simulink model "Ball_and_Plate_MicroLabBox_student"  (R2019b)
settings: Solver=ode1  StartTime=0.0  StopTime=Inf  FixedStep=0.001  RelTol=1e-3
PostLoadFcn:
  | , if any(exist('dsrtsu_mdlpostloadfcn', 'file') ~= 0), dsrtsu_mdlpostloadfcn('Execute', bdroot); end,
InitFcn:
  | , if any(exist('rtifpga_mdlclblib', 'file') ~= 0), rtifpga_mdlclblib('Init', bdroot); end,
undefined symbols (not defined in the file): A_obs, A_robust, B_obs, B_robust, ball_pos_sat, ball_vel_sat, C_obs, C_robust, D_obs, D_robust, g, K_lqr, path, plate_angle_sat, Q_kf, R_kf, Ts_fast, Ts_Inner, Ts_Outer, uA, uB, uC
libraries: rtiemclib x6, simulink x3, rtiethernetlib x3, rti1202lib_dac_class1 x3, mpclib x1
(part 1 of 3)
Description:
  | Standard RTI1202 template.
  | Supported MATLAB version:  R2019b.
settings Model: Tag=RTI1202  DSRTSU_INTERNAL_RTI_VER=570  DSRTSU_INTERNAL_RTI_TYPE=rti1202  RTICANMMDATA=struct('GeneralSetupData',struct('modelroot','C:\git\SystemsAndControlIntegrationProject_5SC25\Experiment\BallANDPlate','generalsettings',struct('filesettings',struct('destfolder',struct('Name','RTICANMM_FILES','Check',1),'buildfolder',struct('Name','.','Check',1),'AbsDestfolder',struct('Name','C:\git\SystemsAndControlIntegrationProject_5SC25\Experiment\BallANDPlate\RTICANMM_FILES'),'AbsBuildfolder',struct('Name','C:\git\SystemsAndControlIntegrationProject_5SC25\Experiment\BallANDPlate'))),'options',struct('addpaths',1,'rmpaths',1,'addtrcexclusion',true,'cannavigator',struct('checkmonitoring',0),'show_usrtrc',0,'use_usrtrc',0),'advanced',struct('options',ones(1,100)),'MPSetup',{{}},'RTI',struct('Type','RTI1202','Ver','7.15','Date','02-Nov-2020'),'modelname','Ball_and_Plate_MicroLabBox_student','block','Ball_and_Plate_MicroLabBox_student'))  DSRTSU_INTERNAL_RTIFPGA=170  Creator=20201603  LastModifiedBy=20242496
settings DataIOCC: ReturnWorkspaceOutputs=off
settings OptimizationCC: BlockReduction=off  OptimizeBlockIOStorage=off  BufferReuse=off  GlobalBufferReuse=off  ExpressionFolding=off  LocalBlockOutputs=off  OptimizeDataStoreBuffers=off  BusAssignmentInplaceUpdate=off
settings DebuggingCC: PregeneratedLibrarySubsystemCodeDiagnostic=none  ArithmeticOperatorsInVariantConditions=warning
settings HardwareCC: ProdBitPerPointer=32  ProdBitPerSizeT=32  ProdBitPerPtrDiffT=32  ProdLargestAtomicInteger=Integer  ProdEndianess=BigEndian  ProdWordSize=32  ProdLongLongMode=on  ProdHWDeviceType=Custom Processor->Custom  TargetIntDivRoundTo=Zero  TargetEndianess=BigEndian  TargetHWDeviceType=Custom Processor->Custom
settings ModelReferenceCC: EnableParallelModelReferenceBuilds=on  ParallelModelReferenceMATLABWorkerInit=Load Top Model
settings SFSimCC: SimUseLocalCustomCode=off  MATLABDynamicMemAlloc=off  CustomCodeUndefinedFunction=UseInterfaceOnly
settings RTWCC: Description=dSPACE DS1202 Hardware Platform  SystemTargetFile=rti1202.tlc  MakeCommand=make_rti  TemplateMakefile=rti1202.tmf  RTWUseLocalCustomCode=off
settings CodeAppCC: StateflowObjectComments=on
settings STFCustomTargetCC: ParMdlRefBuildCompliant=on  SystemTargetFile=rti1202.tlc
settings GRTTargetCC: TargetLangStandard=C89/C90 (ANSI)  CompOptLevelCompliant=off  ConcurrentExecutionCompliant=off  CombineOutputUpdateFcns=off  MatFileLogging=off  CPPClassGenCompliant=off  UseToolchainInfoCompliant=off
settings ConfigComp: CovMetricSettings=dswe

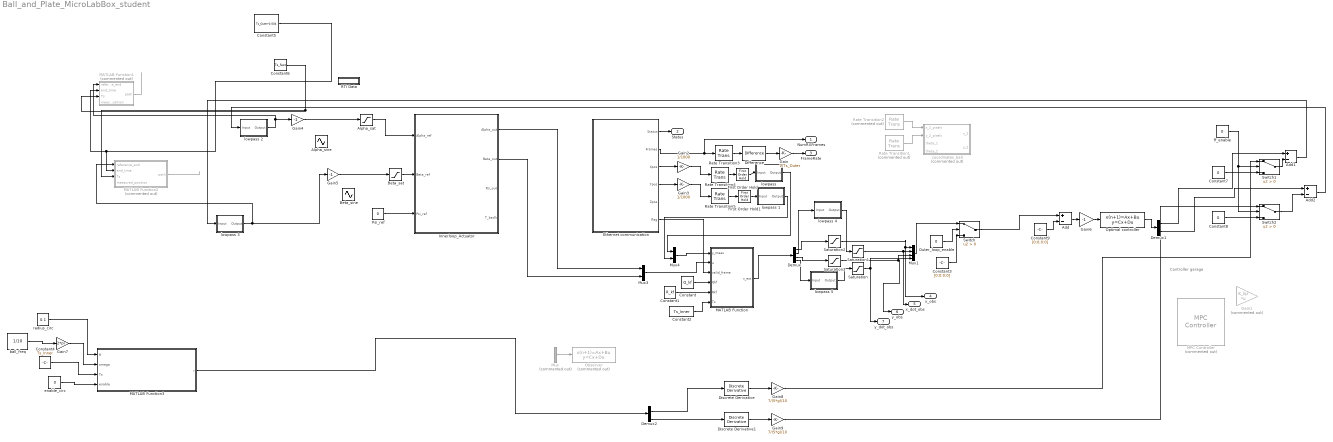
== system Ball_and_Plate_MicroLabBox_student ==
  note: Controller garage
  Add : Sum  Inputs=+-
  Add1 : Sum  Inputs=+-
  Add2 : Sum  Inputs=+-
  "Alpha_sat " : Saturate  UpperLimit=plate_angle_sat  LowerLimit=-plate_angle_sat
  "Alpha_sine " : Sin  Amplitude=0.01  SampleTime=0
  "Beta_sat " : Saturate  UpperLimit=plate_angle_sat  LowerLimit=-plate_angle_sat
  Beta_sine : Sin  Amplitude=0.01  SampleTime=0
  Constant : Constant  Value=Q_kf
  Constant1 : Constant  Value=R_kf
  Constant2 : Constant  Value=Ts_Inner
  Constant3 : Constant  Value=[0;0;0;0]
  Constant4 : Constant  Value=Ts_Inner
  Constant5 : Constant  Value=Ts_Outer-0.004
  Constant6 : Constant  Value=Ts_fast
  Constant7 : Constant  Value=0
  Constant8 : Constant  Value=0
  Constant9 : Constant  Value=[0;0;0;0]
  Demux : Demux
  Demux1 : Demux  Outputs=2
  Demux2 : Demux
  Difference : simulink/Discrete/Difference  ICPrevInput=0  OutMin=[]  OutMax=[]  OutDataType=fixdt(1, 16)  OutScaling=2^-10  DoSatur=off
  Discrete Derivative : simulink/Discrete/Discrete Derivative  gainval=1.0  ICPrevScaledInput=0.0  OutMin=[]  OutMax=[]  OutDataType=fixdt(1, 16)  OutScaling=2^-10  DoSatur=off
  Discrete Derivative1 : simulink/Discrete/Discrete Derivative  gainval=1.0  ICPrevScaledInput=0.0  OutMin=[]  OutMax=[]  OutDataType=fixdt(1, 16)  OutScaling=2^-10  DoSatur=off
  Ethernet communication : Subsystem
  First Order Hold : FirstOrderHold  ErrorTolerance=inf
  First Order Hold1 : FirstOrderHold  ErrorTolerance=inf
  Gain : Gain  Gain=1/Ts_Outer
  Gain1 : Gain  Commented=on  Gain=K_lqr  Multiplication=Matrix(K*u)
  Gain2 : Gain  Gain=1/1000
  Gain3 : Gain  Gain=1/1000
  Gain4 : Gain  Gain=-1
  Gain5 : Gain  Gain=-1
  Gain6 : Gain  Gain=-1
  Gain7 : Gain  Gain=2*pi
  Gain8 : Gain  Gain=7/(5*g)/10
  Gain9 : Gain  Gain=7/(5*g)/10
  Innerloop_Actuator : Subsystem
  MATLAB Function : MATLAB Function  TreatAsAtomicUnit=on
  MATLAB Function1 : MATLAB Function  Commented=on  TreatAsAtomicUnit=on
  MATLAB Function2 : MATLAB Function  Commented=on  TreatAsAtomicUnit=on
  MATLAB Function3 : MATLAB Function  TreatAsAtomicUnit=on
  MPC Controller : mpclib/MPC Controller  Commented=on  SCDEnableBlockLinearizationSpecification=on  mpcobj=mpcobj  is_multiple=0  enable_value=0  return_u0=off  updateMPCinCallerWorkspace=on  md_inport=off  mv_inport=off  uref_inport=off  return_cost=off  return_mvseq=off  return_qpstatus=off  return_xseq=off  return_state=off  return_ovseq=off  state_inport=on  umin_inport=off  umax_inport=off  ymin_inport=off  ymax_inport=off  cc_inport=off  ywt_inport=off  uwt_inport=off  duwt_inport=off  rhoeps_inport=off  pm_inport=off  MaximumP=10  HorizonChoice=FixedHorizon  n_ts=0.02  n_p=25  n_mv=2  n_md=0  n_ud=0  n_mo=4  n_uo=0  BlockDataType=double  SampleTimeInherited=off  switch_inport=off
  Mux : Mux  Commented=on
  Mux1 : Mux
  Mux3 : Mux  Inputs=2
  Mux4 : Mux  Inputs=2
  "Observer " : DiscreteStateSpace  Commented=on  A=A_obs  B=B_obs  C=C_obs  D=D_obs  SampleTime=Ts_Outer
  Optimal controller : DiscreteStateSpace  A=A_robust  B=B_robust  C=C_robust  D=D_robust  SampleTime=Ts_Inner
  Outer_loop_enable : Constant  Value=0
  "Psi_ref " : Constant  Value=0
  RTI Data : Subsystem  Tag=struct('RTIDataServer',struct('RTIDataServerVs','2','RTIModelDescription','struct(''main'',''Ball_and_Plate_MicroLabBox_student'',''sub'','''',''isMp'',0)'))  LoadFcn="if exist('rtidc'), try,  rtidc('DataHostBlockClbLoad', gcbh); catch, disp(['Warning: ''LoadFcn'' for RTI Data block failed: ' lasterr]); end, end,"  mask(RTI_DATA_HOST){}
      mask help:
      | RTI Data Block.
      | This block is used by RTI to store internal model-dependent data.
      | Please keep this block on the root level of the model. Deleting this block will result in data loss.
      |
      | NEVER DELETE OR COPY THIS BLOCK!
      settings: CopyFcn="if exist('rtidc'), try,  rtidc('DataHostBlockClbCopy', gcbh); catch, disp(['Warning: ''CopyFcn'' for RTI Data block failed: ' lasterr]); end, end,"  DeleteFcn="if exist('rtidc'), try,  rtidc('DataHostBlockClbDelete', gcbh); catch, disp(['Warning: ''DeleteFcn'' for RTI Data block failed: ' lasterr]); end, end,"  ModelCloseFcn="if exist('rtidc'), try,  rtidc('DataHostBlockClbModelClose', gcbh); catch, disp(['Warning: ''ModelCloseFcn'' for RTI Data block failed: ' lasterr]); end, end,"  PreSaveFcn="if exist('rtidc'), try,  rtidc('DataHostBlockClbPreSave', gcbh); catch, disp(['Warning: ''PreSaveFcn'' for RTI Data block failed: ' lasterr]); end, end,"  PostSaveFcn="if exist('rtidc'), try,  rtidc('DataHostBlockClbPostSave', gcbh); catch, disp(['Warning: ''PostSaveFcn'' for RTI Data block failed: ' lasterr]); end, end,"  NameChangeFcn="if exist('rtidc'), try,  rtidc('DataHostBlockClbNameChange', gcbh); catch, disp(['Warning: ''NameChangeFcn'' for RTI Data block failed: ' lasterr]); end, end,"
      mask Help:
      | RTI Data Block.
      | This block is used by RTI to store internal model-dependent data.
      | Please keep this block on the root level of the model. Deleting this block will result in data loss.
      | 
      | NEVER DELETE OR COPY THIS BLOCK!
      mask Display:
      | text(0.5, 0.5, 'RTI Data', 'HorizontalAlignment', 'center');
      | plot([1 0]);
  Rate Transition1 : RateTransition  Commented=on  Deterministic=off  OutPortSampleTimeMultiple=Ts_Outer  OutPortSampleTime=Ts_Outer
  Rate Transition2 : RateTransition  Commented=on  Deterministic=off  OutPortSampleTimeMultiple=Ts_Outer  OutPortSampleTime=Ts_Outer
  Rate Transition3 : RateTransition  Deterministic=off  OutPortSampleTimeMultiple=Ts_Outer  OutPortSampleTime=Ts_Outer
  Rate Transition4 : RateTransition  Deterministic=off  OutPortSampleTimeMultiple=Ts_Outer  OutPortSampleTime=Ts_Outer
  Rate Transition5 : RateTransition  Deterministic=off  OutPortSampleTimeMultiple=Ts_Outer  OutPortSampleTime=Ts_Outer
  Saturation : Saturate  UpperLimit=ball_vel_sat  LowerLimit=-ball_vel_sat
  Saturation1 : Saturate  UpperLimit=ball_vel_sat  LowerLimit=-ball_vel_sat
  Saturation2 : Saturate  UpperLimit=ball_pos_sat  LowerLimit=-ball_pos_sat
  Saturation3 : Saturate  UpperLimit=ball_pos_sat  LowerLimit=-ball_pos_sat
  Switch : Switch  Criteria=u2 > Threshold
  Switch1 : Switch  Criteria=u2 > Threshold
  Switch2 : Switch  Criteria=u2 > Threshold
  ball_freq : Constant  Value=1/10
  coordinates_ball : MATLAB Function  Commented=on  TreatAsAtomicUnit=on
  enable_circ : Constant  Value=0
  ff_enable : Constant  Value=0
  "lowpass " : Subsystem
  lowpass 1 : Subsystem
  lowpass 2 : Subsystem
  lowpass 3 : Subsystem
  lowpass 4 : Subsystem
  lowpass 5 : Subsystem
  radius_circ : Constant  Value=0.1
  NumRXFrames : Outport
  Status : Outport  Port=2
  "FrameRate " : Outport  Port=3
  x_obs : Outport  Port=4
  x_dot_obs : Outport  Port=5
  y_obs : Outport  Port=6
  y_dot_obs : Outport  Port=7
  wires:
  Ethernet communication/2("Frames ") -> NumRXFrames/1, Rate Transition3/1
  Rate Transition3/1 -> Difference/1
  Difference/1 -> Gain/1
  Gain/1 -> "FrameRate "/1
  Ethernet communication/1("Status ") -> Status/1
  Rate Transition2/1 -> coordinates_ball/1(x_2_pixels)
  Rate Transition1/1 -> coordinates_ball/2(y_2_pixels)
  "Psi_ref "/1 -> Innerloop_Actuator/3("Psi_ref ")
  Innerloop_Actuator/1(Alpha_out) -> Mux3/1
  Innerloop_Actuator/2(Beta_out) -> Mux3/2
  Mux/1 -> "Observer "/1
  Demux/1 -> Saturation2/1
  Demux/4 -> lowpass 5/1(Input)
  Demux/3 -> Saturation3/1
  Demux/2 -> lowpass 4/1(Input)
  Saturation/1 -> Mux1/4, y_dot_obs/1
  Saturation1/1 -> Mux1/2, x_dot_obs/1
  Mux1/1 -> Switch/1
  Outer_loop_enable/1 -> Switch/2
  Constant3/1 -> Switch/3
  Add1/1 -> lowpass 3/1(Input)
  Add2/1 -> lowpass 2/1(Input)
  "Alpha_sat "/1 -> Innerloop_Actuator/1("Alpha_ref ")
  "Beta_sat "/1 -> Innerloop_Actuator/2("Beta_ref ")
  Ethernet communication/3("Xpos ") -> Gain2/1
  Ethernet communication/4("Ypos ") -> Gain3/1
  Rate Transition4/1 -> First Order Hold/1
  Rate Transition5/1 -> First Order Hold1/1
  Mux3/1 -> MATLAB Function/2(u)
  Mux4/1 -> MATLAB Function/1(y_meas)
  Ethernet communication/6(flag) -> MATLAB Function/3(valid_frame)
  Constant/1 -> MATLAB Function/4(Qkf)
  Constant1/1 -> MATLAB Function/5(Rkf)
  Constant2/1 -> MATLAB Function/6(Ts)
  Gain2/1 -> Rate Transition4/1
  Gain3/1 -> Rate Transition5/1
  "lowpass "/1(Output) -> Mux4/1
  lowpass 1/1(Output) -> Mux4/2
  Gain4/1 -> "Alpha_sat "/1
  Gain5/1 -> "Beta_sat "/1
  Constant5/1 -> MATLAB Function2/2(end_time), MATLAB Function1/2(end_time)
  Constant6/1 -> MATLAB Function2/3(Ts), MATLAB Function1/3(Ts)
  MATLAB Function1/1(path) -> ?
  MATLAB Function2/1(path) -> ?
  lowpass 2/1(Output) -> Gain4/1, MATLAB Function1/1(reference_end)
  lowpass 3/1(Output) -> Gain5/1, MATLAB Function2/1(reference_end)
  lowpass 4/1(Output) -> Saturation1/1
  lowpass 5/1(Output) -> Saturation/1
  Saturation2/1 -> Mux1/1, x_obs/1
  Saturation3/1 -> Mux1/3, y_obs/1
  Switch/1 -> Add/1
  MATLAB Function/1(x_est) -> Demux/1
  First Order Hold/1 -> "lowpass "/1(Input)
  First Order Hold1/1 -> lowpass 1/1(Input)
  Constant4/1 -> MATLAB Function3/3(Ts)
  radius_circ/1 -> MATLAB Function3/1(R)
  ball_freq/1 -> Gain7/1
  Gain7/1 -> MATLAB Function3/2(omega)
  enable_circ/1 -> MATLAB Function3/4(enable)
  MATLAB Function3/1(r) -> Demux2/1
  Demux2/2 -> Discrete Derivative/1
  Demux2/4 -> Discrete Derivative1/1
  Discrete Derivative1/1 -> Gain9/1
  Discrete Derivative/1 -> Gain8/1
  Gain8/1 -> Switch1/1
  Gain9/1 -> Switch2/1
  Demux1/1 -> Add1/1
  Demux1/2 -> Add2/1
  Switch1/1 -> Add1/2
  ff_enable/1 -> Switch2/2, Switch1/2
  Switch2/1 -> Add2/2
  Constant7/1 -> Switch1/3
  Constant8/1 -> Switch2/3
  Constant9/1 -> Add/2
  Add/1 -> Gain6/1
  Optimal controller/1 -> Demux1/1
  Gain6/1 -> Optimal controller/1

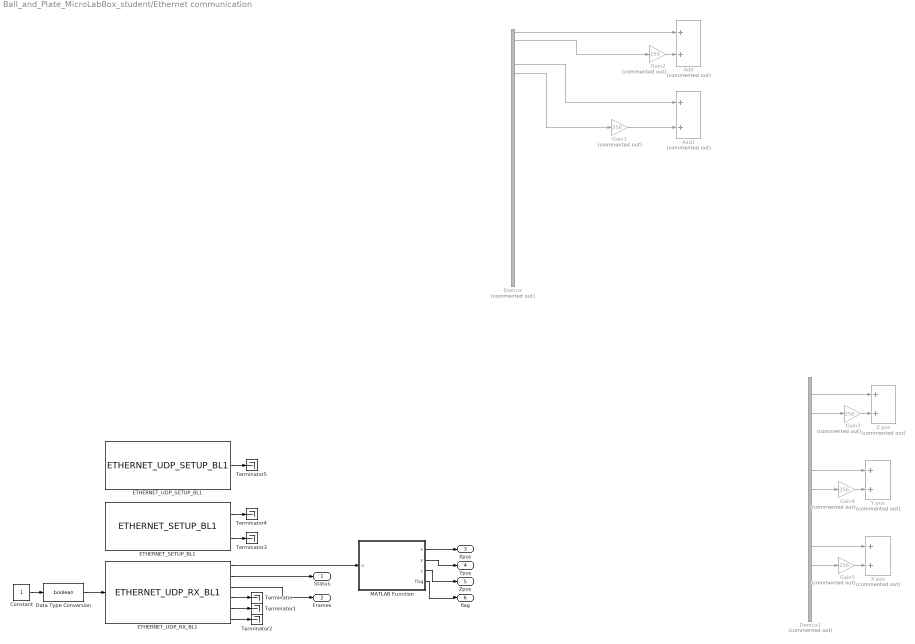
== system Ball_and_Plate_MicroLabBox_student/Ethernet communication ==
  " X pos" : Sum  Commented=on  AccumDataTypeStr=uint16
  Add : Sum  Commented=on  AccumDataTypeStr=uint16
  Add1 : Sum  Commented=on
  Constant : Constant
  Data Type Conversion : DataTypeConversion  OutDataTypeStr=boolean
  Demux : Demux  Commented=on  Outputs=32
  Demux1 : Demux  Commented=on  Outputs=12
  ETHERNET_SETUP_BL1 : rtiethernetlib/ETHERNET_SETUP_BL1  DSProperties=struct('RTI',struct('Version',uint32(2),'BlockType',struct('isSLSource',uint8(0),'isSLSink',uint8(0),'isHWSource',uint8(0),'isHWSink',uint8(0),'isSetup',uint8(1),'isInline',uint8(1),'isNonInline',uint8(0),'isInterrupt',uint8(0),'isChannelwise',uint8(0)),'IOBoardType','DSETHERNET','UnitType','ETHERNET','Identifier','SETUP','DialogType','ML','BlockSet','RTIETHERNET','SlaveProcessor','NONE'))  RTIBlockInterface=struct('OutputPortsWidth',int32([3 1 1 4]),'OutputPortsActive',[1 0 0 1],'OutputPortsName',{{['Link Status'],['Watchdog Status'],['DHCP Status'],['Local IP']}},'OutputPortsDataType',{{'SS_UINT32','SS_UINT32','SS_UINT32','SS_UINT8'}},'InitLevel',3,'IconTransparency','on','BlockDisplay',{{['Ethernet Setup\n\nLocal IP: 192.168.140.8'],'left'}},'DialogFcn','rtiethernetsetupgui','BlockName',struct('Token',{{'ETHERNET_SETUP_BL1'}}))  RTIBlockParameters=struct('DHCPserverMode',{{0,'OFF',[0 1]}},'LocalIpNum1',{{'192','OFF',[0 255]}},'LocalIpNum2',{{'168','OFF',[0 255]}},'LocalIpNum3',{{'140','OFF',[0 255]}},'LocalIpNum4',{{'8','OFF',[0 255]}},'SubnetMaskNum1',{{'255','OFF',[0 255]}},'SubnetMaskNum2',{{'255','OFF',[0 255]}},'SubnetMaskNum3',{{'255','OFF',[0 255]}},'SubnetMaskNum4',{{'0','OFF',[0 255]}},'GatewayNum1',{{'0','OFF',[0 255]}},'GatewayNum2',{{'0','OFF',[0 255]}},'GatewayNum3',{{'0','OFF',[0 255]}},'GatewayNum4',{{'0','OFF',[0 255]}},'LinkStatusOutPortMode',{{1,'OFF',[0 1]}},'NumOfEthConnectors',{{3,'ON',[1 16]}},'WatchdogStatusOutPortMode',{{0,'OFF',[0 1]}},'LocalIpOutPortMode',{{1,'OFF',[0 1]}},'IpAndSubmaskCheck',{{int32(1),'OFF',[0 1]}},'TLCFileName',{{'rtiethernetsetup','OFF',[]}})  RTISFcnParameters=struct('DHCPserverMode','int32','LocalIpNum1','uint8','LocalIpNum2','uint8','LocalIpNum3','uint8','LocalIpNum4','uint8','SubnetMaskNum1','uint8','SubnetMaskNum2','uint8','SubnetMaskNum3','uint8','SubnetMaskNum4','uint8','GatewayNum1','uint8','GatewayNum2','uint8','GatewayNum3','uint8','GatewayNum4','uint8','LinkStatusOutPortMode','int32','NumOfEthConnectors','int32','WatchdogStatusOutPortMode','int32','LocalIpOutPortMode','int32','TLCFileName','char')  RTIBlockParaDefault=struct('DHCPserverMode',0,'LocalIpNum1',192,'LocalIpNum2',168,'LocalIpNum3',140,'LocalIpNum4',6,'SubnetMaskNum1',255,'SubnetMaskNum2',255,'SubnetMaskNum3',255,'SubnetMaskNum4',0,'GatewayNum1',0,'GatewayNum2',0,'GatewayNum3',0,'GatewayNum4',0,'LinkStatusOutPortMode',1,'NumOfEthConnectors',3,'WatchdogStatusOutPortMode',0,'LocalIpOutPortMode',0,'IpAndSubmaskCheck',1,'TLCFileName','rtiethernetsetup')
      settings: SourceProductName=dSPACE RTI Ethernet Blockset
  ETHERNET_UDP_RX_BL1 : rtiethernetlib/ETHERNET_UDP_RX_BL1  DSProperties=struct('RTI',struct('Version',uint32(1),'BlockType',struct('isSLSource',uint8(1),'isSLSink',uint8(1),'isHWSource',uint8(0),'isHWSink',uint8(1),'isSetup',uint8(0),'isInline',uint8(1),'isNonInline',uint8(0),'isInterrupt',uint8(0),'isChannelwise',uint8(0)),'IOBoardType','DSETHERNET','UnitType','UDP','Identifier','RXUDP','DialogType','ML','BlockSet','RTIETHERNET','SlaveProcessor','NONE'))  RTIBlockInterface=struct('OutputPortsWidth',int32([12 1 1 1 4 1]),'OutputPortsActive',[1 1 1 1 1 1],'OutputPortsName',{{'Data','Status',['Received Frames'],['Received Bytes'],['Remote IP'],['Remote Port']}},'OutputPortsDataType',{{'SS_UINT8','SS_UINT32','SS_DOUBLE','SS_UINT32','SS_UINT8','SS_UINT16'}},'InputPortsWidth',int32(1),'InputPortsActive',1,'InputPortsName',{{'Enable'}},'InputPortsDataType',{{'SS_BOOLEAN'}},'RWork',{{{'RECEIVED_FRAMES',uint32(1)}}},'InitLevel',3,'IconTransparency','on','BlockDisplay',{{['Ethernet UDP/IP\nRX\n\nSocket ID: 1'],'center'}},'DialogFcn','rtiethernetrxudpgui','BlockName',struct('Token',{{'ETHERNET_UDP_RX_BL1'}}))  RTIBlockParameters=struct('SocketIdIndex',{{2,'OFF',[1 2]}},'SocketId',{{1,'OFF',[-1 inf]}},'RemoteIp',{{['<NOT AVAILABLE>'],'OFF',[]}},'RemotePort',{{['<NOT AVAILABLE>'],'OFF',[]}},'LocalPort',{{49001,'OFF',[]}},'FrameSize',{{'12','OFF',[1 65507]}},'EnableVariableFrameSize',{{1,'OFF',[0 1]}},'VariableFrameSizeMode',{{1,'OFF',[1 2]}},'InterruptMode',{{0,'OFF',[0 1]}},'RemoteIpOutPortMode',{{1,'OFF',[0 1]}},'RemotePortOutPortMode',{{1,'OFF',[0 1]}},'TLCFileName',{{'rtiethernetrxudp','OFF',[]}})  RTISFcnParameters=struct('SocketIdIndex','int32','SocketId','double','FrameSize','uint16','EnableVariableFrameSize','int32','VariableFrameSizeMode','int32','InterruptMode','int32','RemoteIpOutPortMode','int32','RemotePortOutPortMode','int32','TLCFileName','char')  RTIBlockParaDefault=struct('SocketIdIndex',1,'SocketId',-1,'RemoteIp',['<NOT AVAILABLE>'],'RemotePort',['<NOT AVAILABLE>'],'LocalPort',['<NOT AVAILABLE>'],'FrameSize',1024,'EnableVariableFrameSize',0,'VariableFrameSizeMode',1,'InterruptMode',0,'RemoteIpOutPortMode',0,'RemotePortOutPortMode',0,'TLCFileName','rtiethernetrxudp')
      settings: SourceProductName=dSPACE RTI Ethernet Blockset
  ETHERNET_UDP_SETUP_BL1 : rtiethernetlib/ETHERNET_UDP_SETUP_BL1  DSProperties=struct('RTI',struct('Version',uint32(2),'BlockType',struct('isSLSource',uint8(1),'isSLSink',uint8(1),'isHWSource',uint8(0),'isHWSink',uint8(0),'isSetup',uint8(0),'isInline',uint8(1),'isNonInline',uint8(0),'isInterrupt',uint8(0),'isChannelwise',uint8(0)),'IOBoardType','DSETHERNET','UnitType','UDP','Identifier','SETUPUDP','DialogType','ML','BlockSet','RTIETHERNET','SlaveProcessor','NONE'))  RTIBlockInterface=struct('OutputPortsWidth',int32(2),'OutputPortsActive',1,'OutputPortsName',{{['RX Dropped Frames']}},'OutputPortsDataType',{{'SS_DOUBLE'}},'InputPortsWidth',int32([4 1]),'InputPortsActive',int32([0 0]),'InputPortsName',{{['RX Remote IP Filter'],['RX Remote Port Filter']}},'InputPortsDataType',{{'SS_UINT8','SS_UINT16'}},'RWork',{{{'RX_DROPPED_FRAMES',uint32(2)}}},'InitLevel',3,'IconTransparency','on','BlockDisplay',{{['Ethernet UDP/IP\nSetup\n\nSocket ID: 1'],'center'}},'DialogFcn','rtiethernetsetupudpgui','BlockName',struct('Token',{{'ETHERNET_UDP_SETUP_BL1'}}))  RTIBlockParameters=struct('SocketId',{{1,'OFF',[]}},'EnableSocketBind',{{1,'OFF',[0 1]}},'AcceptAnyRxRemoteIp',{{1,'OFF',[0 1]}},'RxRemoteIpNum1',{{'192','OFF',[0 255]}},'RxRemoteIpNum2',{{'168','OFF',[0 255]}},'RxRemoteIpNum3',{{'140','OFF',[0 255]}},'RxRemoteIpNum4',{{'100','OFF',[0 255]}},'EnableDynamicRxRemoteIpFilter',{{0,'OFF',[0 1]}},'AcceptAnyRxRemotePort',{{1,'OFF',[0 1]}},'RxRemotePort',{{'57272','OFF',[1 65535]}},'EnableDynamicRxRemotePortFilter',{{0,'OFF',[0 1]}},'TxRemoteIpNum1',{{'192','OFF',[0 255]}},'TxRemoteIpNum2',{{'168','OFF',[0 255]}},'TxRemoteIpNum3',{{'140','OFF',[0 255]}},'TxRemoteIpNum4',{{'100','OFF',[0 255]}},'TxRemotePort',{{'49002','OFF',[1 65535]}},'SpecifyLocalPort',{{1,'OFF',[0 1]}},'LocalPort',{{'49001','OFF',[1 65535]}},'InterruptMode',{{0,'OFF',[0 1]}},'RxDroppedFramesOutPortMode',{{1,'OFF',[0 1]}},'RemoteIpNumCheck',{{0,'OFF',[0 1]}},'RemotePortCheck',{{0,'OFF',[0 1]}},'LocalPortCheck',{{1,'OFF',[0 1]}},'DHCPserverModeEnabled',{{0,'OFF',[0 1]}},'TLCFileName',{{'rtiethernetsetupudp','OFF',[]}})  RTISFcnParameters=struct('SocketId','double','EnableSocketBind','int32','AcceptAnyRxRemoteIp','int32','RxRemoteIpNum1','uint8','RxRemoteIpNum2','uint8','RxRemoteIpNum3','uint8','RxRemoteIpNum4','uint8','EnableDynamicRxRemoteIpFilter','int32','AcceptAnyRxRemotePort','int32','RxRemotePort','uint16','EnableDynamicRxRemotePortFilter','int32','TxRemoteIpNum1','uint8','TxRemoteIpNum2','uint8','TxRemoteIpNum3','uint8','TxRemoteIpNum4','uint8','TxRemotePort','uint16','SpecifyLocalPort','int32','LocalPort','uint16','InterruptMode','int32','RxDroppedFramesOutPortMode','int32','DHCPserverModeEnabled','int32','TLCFileName','char')  RTIBlockParaDefault=struct('SocketId',-1,'EnableSocketBind',1,'AcceptAnyRxRemoteIp',1,'RxRemoteIpNum1',0,'RxRemoteIpNum2',0,'RxRemoteIpNum3',0,'RxRemoteIpNum4',0,'EnableDynamicRxRemoteIpFilter',0,'AcceptAnyRxRemotePort',1,'RxRemotePort',49002,'EnableDynamicRxRemotePortFilter',0,'TxRemoteIpNum1',0,'TxRemoteIpNum2',0,'TxRemoteIpNum3',0,'TxRemoteIpNum4',0,'TxRemotePort',49002,'SpecifyLocalPort',0,'LocalPort',49001,'InterruptMode',0,'RxDroppedFramesOutPortMode',0,'RemoteIpNumCheck',0,'RemotePortCheck',0,'LocalPortCheck',0,'DHCPserverModeEnabled',0,'TLCFileName','rtiethernetsetupudp')
      settings: SourceProductName=dSPACE RTI Ethernet Blockset
  Gain{1..5} (5 alike) : Gain  Commented=on  Gain=256  OutDataTypeStr=uint16
  MATLAB Function : MATLAB Function  TreatAsAtomicUnit=on
  Terminator{,1..5} (6 alike) : Terminator
  Y pos : Sum  Commented=on  AccumDataTypeStr=uint16
  Z pos : Sum  Commented=on  AccumDataTypeStr=uint16
  "Status " : Outport
  "Frames " : Outport  Port=2
  "Xpos " : Outport  Port=3
  "Ypos " : Outport  Port=4
  Zpos : Outport  Port=5
  flag : Outport  Port=6
  wires:
  Demux/1 -> Add/1
  Data Type Conversion/1 -> ETHERNET_UDP_RX_BL1/1
  ETHERNET_UDP_RX_BL1/4 -> Terminator/1
  Demux/2 -> Gain2/1
  Gain1/1 -> Add1/2
  Demux/5 -> Add1/1
  Demux/6 -> Gain1/1
  ETHERNET_UDP_RX_BL1/3 -> "Frames "/1
  Constant/1 -> Data Type Conversion/1
  Gain2/1 -> Add/2
  ETHERNET_UDP_RX_BL1/2 -> "Status "/1
  ETHERNET_SETUP_BL1/1 -> Terminator4/1
  ETHERNET_UDP_RX_BL1/5 -> Terminator1/1
  ETHERNET_UDP_RX_BL1/6 -> Terminator2/1
  ETHERNET_SETUP_BL1/2 -> Terminator3/1
  ETHERNET_UDP_SETUP_BL1/1 -> Terminator5/1
  Gain3/1 -> Z pos/2
  Demux1/1 -> Z pos/1
  Demux1/2 -> Gain3/1
  Gain4/1 -> Y pos/2
  Demux1/5 -> Y pos/1
  Demux1/6 -> Gain4/1
  Gain5/1 -> " X pos"/2
  Demux1/9 -> " X pos"/1
  Demux1/10 -> Gain5/1
  ETHERNET_UDP_RX_BL1/1 -> MATLAB Function/1(u)
  MATLAB Function/2(y) -> "Ypos "/1
  MATLAB Function/1(x) -> "Xpos "/1
  MATLAB Function/3(z) -> Zpos/1
  MATLAB Function/4(flag) -> flag/1

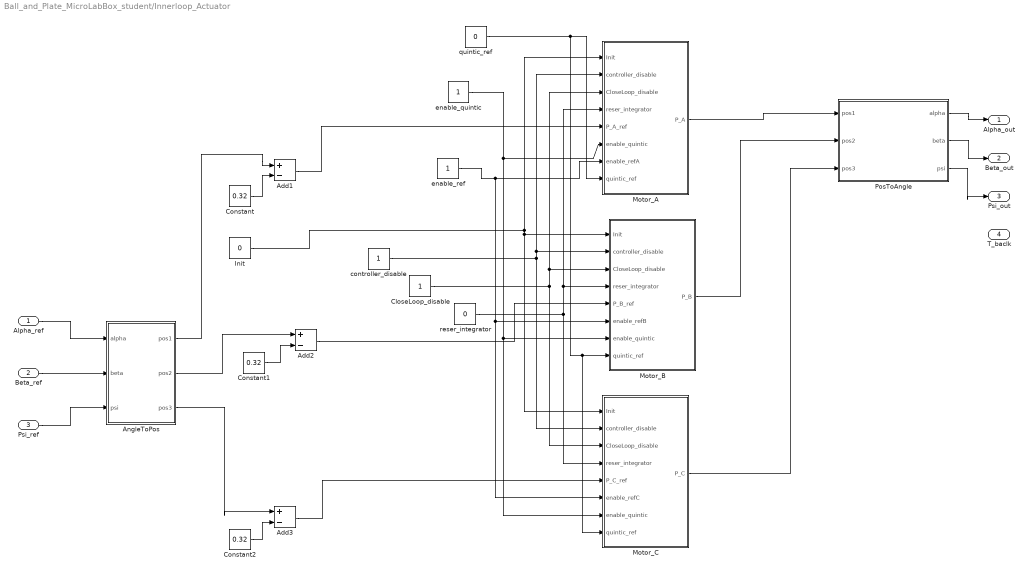
== system Ball_and_Plate_MicroLabBox_student/Innerloop_Actuator ==
  "Alpha_ref " : Inport
  "Beta_ref " : Inport  Port=2
  "Psi_ref " : Inport  Port=3
  Add1 : Sum  Inputs=+-
  Add2 : Sum  Inputs=+-
  Add3 : Sum  Inputs=+-
  "AngleToPos " : MATLAB Function  TreatAsAtomicUnit=on
  CloseLoop_disable : Constant
  Constant : Constant  Value=0.32
  Constant1 : Constant  Value=0.32
  Constant2 : Constant  Value=0.32
  "Init " : Constant  Value=0
  Motor_A : Subsystem
  Motor_B : Subsystem
  Motor_C : Subsystem
  "PosToAngle " : MATLAB Function  TreatAsAtomicUnit=on
  controller_disable : Constant
  "enable_quintic " : Constant
  "enable_ref " : Constant
  "quintic_ref " : Constant  Value=0
  reser_integrator : Constant  Value=0
  Alpha_out : Outport
  Beta_out : Outport  Port=2
  Psi_out : Outport  Port=3
  T_baclk : Outport  Port=4
  wires:
  Motor_C/1(P_C) -> "PosToAngle "/3(pos3)
  Add2/1 -> Motor_B/5(P_B_ref)
  CloseLoop_disable/1 -> Motor_A/3(CloseLoop_disable), Motor_B/3(CloseLoop_disable), Motor_C/3(CloseLoop_disable)
  Constant/1 -> Add1/2
  Constant2/1 -> Add3/2
  Constant1/1 -> Add2/2
  controller_disable/1 -> Motor_A/2(controller_disable), Motor_B/2(controller_disable), Motor_C/2(controller_disable)
  Add3/1 -> Motor_C/5(P_C_ref)
  "Init "/1 -> Motor_B/1(Init), Motor_C/1(Init), Motor_A/1(Init)
  reser_integrator/1 -> Motor_A/4(reser_integrator), Motor_B/4(reser_integrator), Motor_C/4(reser_integrator)
  Add1/1 -> Motor_A/5(P_A_ref)
  Motor_B/1(P_B) -> "PosToAngle "/2(pos2)
  "AngleToPos "/1(pos1) -> Add1/1
  "Alpha_ref "/1 -> "AngleToPos "/1(alpha)
  "Beta_ref "/1 -> "AngleToPos "/2(beta)
  "Psi_ref "/1 -> "AngleToPos "/3(psi)
  "AngleToPos "/2(pos2) -> Add2/1
  "AngleToPos "/3(pos3) -> Add3/1
  "enable_quintic "/1 -> Motor_B/7("enable_quintic "), Motor_C/7("enable_quintic "), Motor_A/6("enable_quintic ")
  "enable_ref "/1 -> Motor_C/6(enable_refC), Motor_B/6("enable_refB "), Motor_A/7("enable_refA ")
  "quintic_ref "/1 -> Motor_A/8(quintic_ref), Motor_C/8(quintic_ref), Motor_B/8(quintic_ref)
  "PosToAngle "/3(psi) -> Psi_out/1
  "PosToAngle "/2(beta) -> Beta_out/1
  "PosToAngle "/1(alpha) -> Alpha_out/1
  Motor_A/1(P_A) -> "PosToAngle "/1(pos1)

== system Ball_and_Plate_MicroLabBox_student/RTI Data ==
  RTI Data Store : Subsystem  Tag="struct('public',struct('sub',struct('name',{{'Ball_and_Plate_MicroLabBox_student'}},'data',{{struct('TH',struct('thTaskInfo',struct('taskType',{'TIMER','HWINT','TMRINT','SWINT','GLINT'},'tasksNumOf',{1,0,0,0,0},'srcIds',{{'TIMERA'},{},{},{},{}},'taskNames',{{['Timer Task 1']},{},{},{},{}})),'th_tc',struct('dataType','TASK','taskGroupId','','taskGroupList',{{}},'taskSchedulingPolicy','FCFS','taskType','TIMER','blkh',-1,'srcId','TIMERA','srcSgnName',['Timer A interrupt'],'srcCpuName','','taskName',['Timer Task 1  [0.001] s'],'taskNameDisplayExt','','smplTime',0.001,'smplTimeOffs',0,'hasFixedPriority',0,'priority',1,'hasFixedOvc',0,'ovcType',1,'ovcMax',1),'tc_th',struct('dataType','TASK','taskGroupId','','taskGroupList',{{}},'taskSchedulingPolicy','FCFS','taskType','TIMER','blkh',-1,'srcId','TIMERA','srcSgnName',['Timer A interrupt'],'srcCpuName','','taskName',['Timer Task 1  [0.001] s'],'taskNameDisplayExt','','smplTime',0.001,'smplTimeOffs',0,'hasFixedPriority',0,'priority',1,'hasFixedOvc',0,'ovcType',1,'ovcMax',1))}})),'private',struct('version',struct('dsVer',uint32(2)),'access',struct('modified',['16-Jun-2026 16:38:03'],'type','Model','isPerm',1)))"  mask(RTI_DATA_STORE){}
      mask help:
      | RTI Data Store Block. This block is used by RTI to store internal model dependent data. Deleting this block will result in data loss.
      |
      | NEVER DELETE, COPY, OR MODIFY THIS BLOCK!
      mask Help:
      | RTI Data Store Block. This block is used by RTI to store internal model dependent data. Deleting this block will result in data loss.
      | 
      | NEVER DELETE, COPY, OR MODIFY THIS BLOCK!
      mask Display: text(0.5, 0.5, ' ', 'HorizontalAlignment', 'center');

== system Ball_and_Plate_MicroLabBox_student/lowpass  ==
  Input : Inport
  Dct1lowpass2 : S-Function  FunctionName=dlowpass1  Parameters=f_den, 0.001  SFunctionDeploymentMode=off  EnableBusSupport=off  mask(dctools){f_den=30}
      mask prompts: f_den "Pole [Hz]"
      mask help: This block implements a discrete time 1st order lowpass filter.
      mask Display: disp('DCT 1st order lowpass')
  Gain1 : Gain  SaturateOnIntegerOverflow=on  OutDataTypeStr=Inherit: Same as input  ParamDataTypeStr=Inherit: Same as input
  Output : Outport
  wires:
  Input/1 -> Gain1/1
  Gain1/1 -> Dct1lowpass2/1
  Dct1lowpass2/1 -> Output/1

== system Ball_and_Plate_MicroLabBox_student/lowpass 1 ==
  Input : Inport
  Dct1lowpass2 : S-Function  FunctionName=dlowpass1  Parameters=f_den, 0.001  SFunctionDeploymentMode=off  EnableBusSupport=off  mask(dctools){f_den=30}
      mask prompts: f_den "Pole [Hz]"
      mask help: This block implements a discrete time 1st order lowpass filter.
      mask Display: disp('DCT 1st order lowpass')
  Gain1 : Gain  SaturateOnIntegerOverflow=on  OutDataTypeStr=Inherit: Same as input  ParamDataTypeStr=Inherit: Same as input
  Output : Outport
  wires:
  Input/1 -> Gain1/1
  Gain1/1 -> Dct1lowpass2/1
  Dct1lowpass2/1 -> Output/1

== system Ball_and_Plate_MicroLabBox_student/lowpass 2 ==
  Input : Inport
  Dct1lowpass2 : S-Function  FunctionName=dlowpass1  Parameters=f_den, 0.001  SFunctionDeploymentMode=off  EnableBusSupport=off  mask(dctools){f_den=25}
      mask prompts: f_den "Pole [Hz]"
      mask help: This block implements a discrete time 1st order lowpass filter.
      mask Display: disp('DCT 1st order lowpass')
  Gain1 : Gain  SaturateOnIntegerOverflow=on  OutDataTypeStr=Inherit: Same as input  ParamDataTypeStr=Inherit: Same as input
  Output : Outport
  wires:
  Input/1 -> Gain1/1
  Gain1/1 -> Dct1lowpass2/1
  Dct1lowpass2/1 -> Output/1

== system Ball_and_Plate_MicroLabBox_student/lowpass 3 ==
  Input : Inport
  Dct1lowpass2 : S-Function  FunctionName=dlowpass1  Parameters=f_den, 0.001  SFunctionDeploymentMode=off  EnableBusSupport=off  mask(dctools){f_den=25}
      mask prompts: f_den "Pole [Hz]"
      mask help: This block implements a discrete time 1st order lowpass filter.
      mask Display: disp('DCT 1st order lowpass')
  Gain1 : Gain  SaturateOnIntegerOverflow=on  OutDataTypeStr=Inherit: Same as input  ParamDataTypeStr=Inherit: Same as input
  Output : Outport
  wires:
  Input/1 -> Gain1/1
  Gain1/1 -> Dct1lowpass2/1
  Dct1lowpass2/1 -> Output/1

== system Ball_and_Plate_MicroLabBox_student/lowpass 4 ==
  Input : Inport
  Dct1lowpass2 : S-Function  FunctionName=dlowpass1  Parameters=f_den, 0.001  SFunctionDeploymentMode=off  EnableBusSupport=off  mask(dctools){f_den=50}
      mask prompts: f_den "Pole [Hz]"
      mask help: This block implements a discrete time 1st order lowpass filter.
      mask Display: disp('DCT 1st order lowpass')
  Gain1 : Gain  SaturateOnIntegerOverflow=on  OutDataTypeStr=Inherit: Same as input  ParamDataTypeStr=Inherit: Same as input
  Output : Outport
  wires:
  Input/1 -> Gain1/1
  Gain1/1 -> Dct1lowpass2/1
  Dct1lowpass2/1 -> Output/1

== system Ball_and_Plate_MicroLabBox_student/lowpass 5 ==
  Input : Inport
  Dct1lowpass2 : S-Function  FunctionName=dlowpass1  Parameters=f_den, 0.001  SFunctionDeploymentMode=off  EnableBusSupport=off  mask(dctools){f_den=50}
      mask prompts: f_den "Pole [Hz]"
      mask help: This block implements a discrete time 1st order lowpass filter.
      mask Display: disp('DCT 1st order lowpass')
  Gain1 : Gain  SaturateOnIntegerOverflow=on  OutDataTypeStr=Inherit: Same as input  ParamDataTypeStr=Inherit: Same as input
  Output : Outport
  wires:
  Input/1 -> Gain1/1
  Gain1/1 -> Dct1lowpass2/1
  Dct1lowpass2/1 -> Output/1

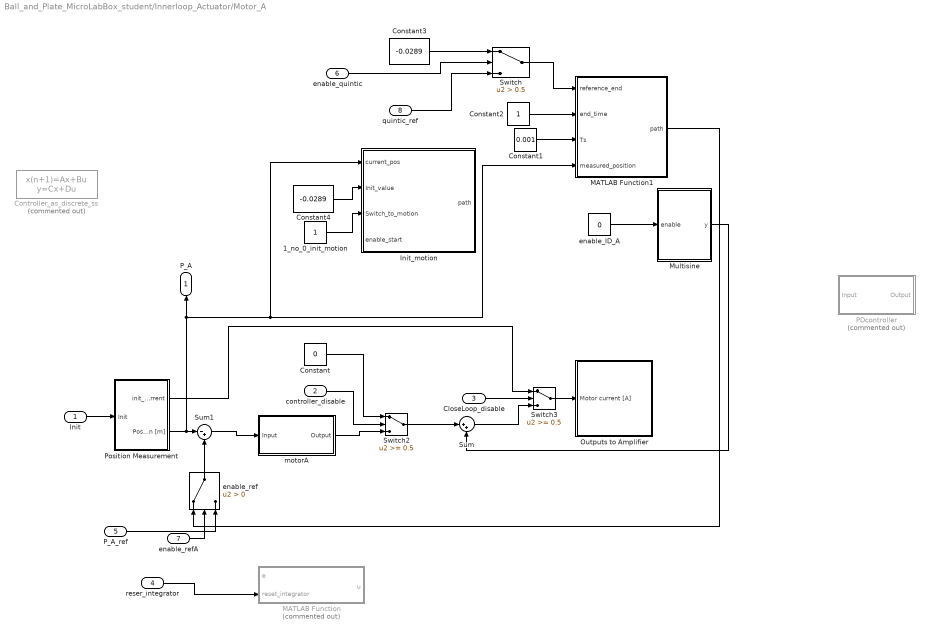
== system Ball_and_Plate_MicroLabBox_student/Innerloop_Actuator/Motor_A ==
  Init : Inport
  controller_disable : Inport  Port=2
  CloseLoop_disable : Inport  Port=3
  reser_integrator : Inport  Port=4
  P_A_ref : Inport  Port=5
  "enable_quintic " : Inport  Port=6
  "enable_refA " : Inport  Port=7
  quintic_ref : Inport  Port=8
  1_no_0_init_motion : Constant
  Constant : Constant  Value=0
  Constant1 : Constant  Value=0.001
  Constant2 : Constant
  Constant3 : Constant  Value=-0.0289
  Constant4 : Constant  Value=-0.0289
  Controller_as_discrete_ss : DiscreteStateSpace  Commented=on  A=[0.5498,0.8818;0,0.8543]  B=[5.1803;10.8938]  C=[-5.1480,10.8259]  D=63.6008  SampleTime=-1
  Init_motion : Subsystem
  MATLAB Function : MATLAB Function  Commented=on  TreatAsAtomicUnit=on
  MATLAB Function1 : MATLAB Function  TreatAsAtomicUnit=on
  Multisine : Subsystem
  Outputs to Amplifier : Subsystem  TreatAsAtomicUnit=on
  PDcontroller : Subsystem  Commented=on
  Position Measurement : Subsystem  TreatAsAtomicUnit=on
  Sum : Sum  Inputs=|++
  Sum1 : Sum  Inputs=|-+  SaturateOnIntegerOverflow=on
  Switch : Switch  Criteria=u2 > Threshold  Threshold=0.5
  Switch2 : Switch  Threshold=0.5
  Switch3 : Switch  Threshold=0.5
  "enable_ID_A " : Constant  Value=0
  "enable_ref " : Switch  Criteria=u2 > Threshold
  "motorA " : Subsystem
  P_A : Outport
  wires:
  "motorA "/1(Output) -> Switch2/3
  Switch3/1 -> Outputs to Amplifier/1(Motor current [A])
  Position Measurement/2(Position [m]) -> MATLAB Function1/4(measured_position), Init_motion/1(current_pos), P_A/1, Sum1/1
  Position Measurement/1(init_current) -> Switch3/1
  CloseLoop_disable/1 -> Switch3/2
  reser_integrator/1 -> MATLAB Function/2(reset_integrator)
  Sum1/1 -> "motorA "/1(Input)
  Constant/1 -> Switch2/1
  controller_disable/1 -> Switch2/2
  P_A_ref/1 -> "enable_ref "/3
  Init/1 -> Position Measurement/1(Init)
  Constant4/1 -> Init_motion/2(Init_value)
  1_no_0_init_motion/1 -> Init_motion/3(Switch_to_motion)
  "enable_ID_A "/1 -> Multisine/1(enable)
  Switch2/1 -> Sum/1
  Sum/1 -> Switch3/3
  Multisine/1(y) -> Sum/2
  "enable_ref "/1 -> Sum1/2
  "enable_refA "/1 -> "enable_ref "/2
  Constant1/1 -> MATLAB Function1/3(Ts)
  Constant2/1 -> MATLAB Function1/2(end_time)
  Constant3/1 -> Switch/1
  Switch/1 -> MATLAB Function1/1(reference_end)
  quintic_ref/1 -> Switch/3
  "enable_quintic "/1 -> Switch/2
  MATLAB Function1/1(path) -> "enable_ref "/1

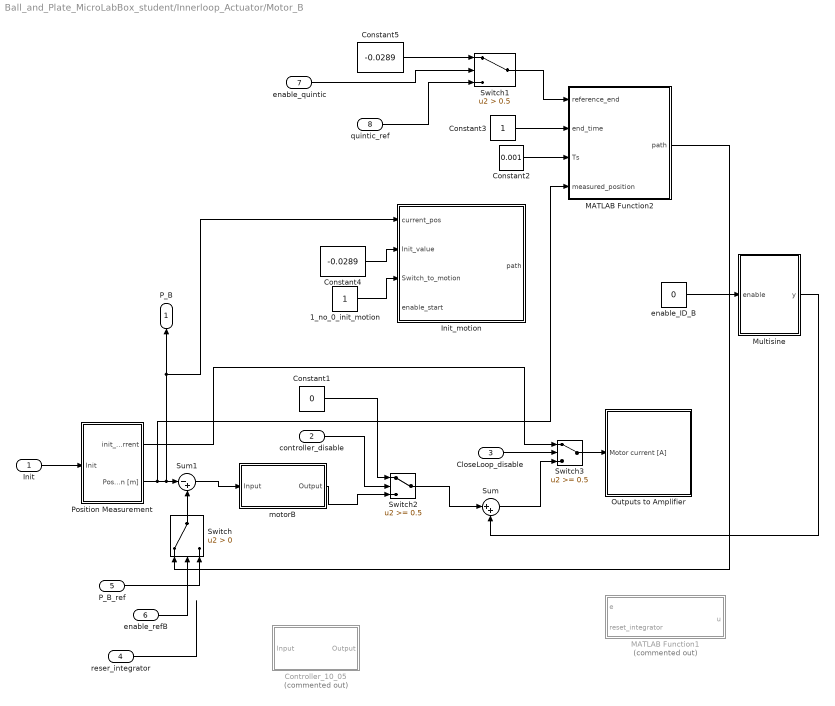
== system Ball_and_Plate_MicroLabBox_student/Innerloop_Actuator/Motor_B ==
  Init : Inport
  controller_disable : Inport  Port=2
  CloseLoop_disable : Inport  Port=3
  reser_integrator : Inport  Port=4
  P_B_ref : Inport  Port=5
  "enable_refB " : Inport  Port=6
  "enable_quintic " : Inport  Port=7
  quintic_ref : Inport  Port=8
  1_no_0_init_motion : Constant
  Constant1 : Constant  Value=0
  Constant2 : Constant  Value=0.001
  Constant3 : Constant
  Constant4 : Constant  Value=-0.0289
  Constant5 : Constant  Value=-0.0289
  Controller_10_05 : Subsystem  Commented=on
  Init_motion : Subsystem
  MATLAB Function1 : MATLAB Function  Commented=on  TreatAsAtomicUnit=on
  MATLAB Function2 : MATLAB Function  TreatAsAtomicUnit=on
  Multisine : Subsystem
  Outputs to Amplifier : Subsystem  TreatAsAtomicUnit=on
  Position Measurement : Subsystem  TreatAsAtomicUnit=on
  Sum : Sum  Inputs=|++
  Sum1 : Sum  Inputs=|-+  SaturateOnIntegerOverflow=on
  Switch : Switch  Criteria=u2 > Threshold
  Switch1 : Switch  Criteria=u2 > Threshold  Threshold=0.5
  Switch2 : Switch  Threshold=0.5
  Switch3 : Switch  Threshold=0.5
  "enable_ID_B " : Constant  Value=0
  motorB : Subsystem
  P_B : Outport
  wires:
  motorB/1(Output) -> Switch2/3
  Switch3/1 -> Outputs to Amplifier/1(Motor current [A])
  Position Measurement/2(Position [m]) -> MATLAB Function2/4(measured_position), Init_motion/1(current_pos), P_B/1, Sum1/1
  Position Measurement/1(init_current) -> Switch3/1
  Switch2/1 -> Sum/1
  CloseLoop_disable/1 -> Switch3/2
  Sum1/1 -> motorB/1(Input)
  controller_disable/1 -> Switch2/2
  Constant1/1 -> Switch2/1
  Init/1 -> Position Measurement/1(Init)
  reser_integrator/1 -> ?
  "enable_ID_B "/1 -> Multisine/1(enable)
  Sum/1 -> Switch3/3
  Multisine/1(y) -> Sum/2
  Constant4/1 -> Init_motion/2(Init_value)
  1_no_0_init_motion/1 -> Init_motion/3(Switch_to_motion)
  Switch/1 -> Sum1/2
  P_B_ref/1 -> Switch/3
  "enable_refB "/1 -> Switch/2
  Constant3/1 -> MATLAB Function2/2(end_time)
  Switch1/1 -> MATLAB Function2/1(reference_end)
  Constant2/1 -> MATLAB Function2/3(Ts)
  MATLAB Function2/1(path) -> Switch/1
  quintic_ref/1 -> Switch1/3
  Constant5/1 -> Switch1/1
  "enable_quintic "/1 -> Switch1/2

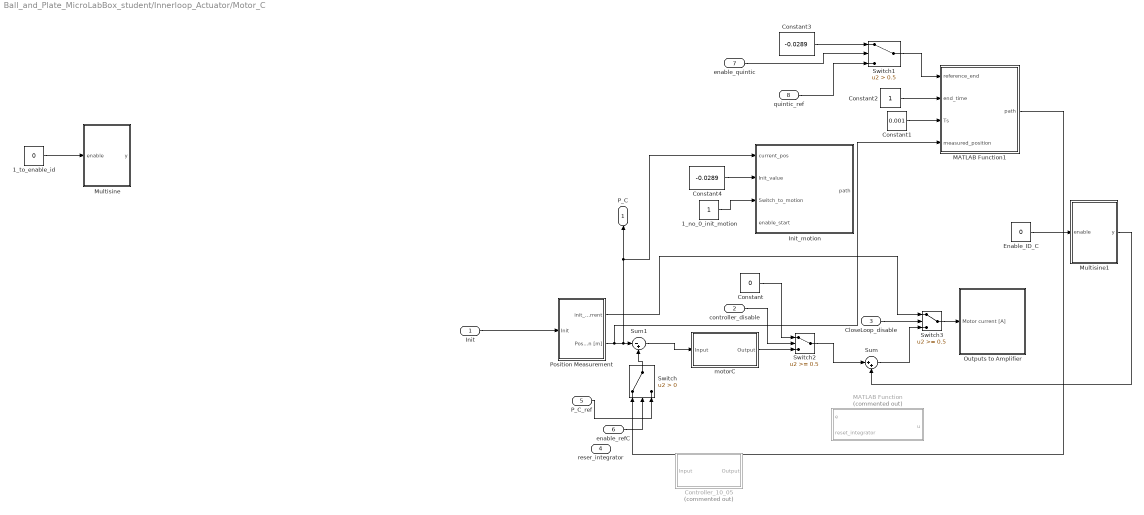
== system Ball_and_Plate_MicroLabBox_student/Innerloop_Actuator/Motor_C ==
  Init : Inport
  controller_disable : Inport  Port=2
  CloseLoop_disable : Inport  Port=3
  reser_integrator : Inport  Port=4
  P_C_ref : Inport  Port=5
  enable_refC : Inport  Port=6
  "enable_quintic " : Inport  Port=7
  quintic_ref : Inport  Port=8
  1_no_0_init_motion : Constant
  1_to_enable_id : Constant  Value=0
  Constant : Constant  Value=0
  Constant1 : Constant  Value=0.001
  Constant2 : Constant
  Constant3 : Constant  Value=-0.0289
  Constant4 : Constant  Value=-0.0289
  Controller_10_05 : Subsystem  Commented=on
  "Enable_ID_C " : Constant  Value=0
  Init_motion : Subsystem
  MATLAB Function : MATLAB Function  Commented=on  TreatAsAtomicUnit=on
  MATLAB Function1 : MATLAB Function  TreatAsAtomicUnit=on
  Multisine : Subsystem
  Multisine1 : Subsystem
  Outputs to Amplifier : Subsystem  TreatAsAtomicUnit=on
  Position Measurement : Subsystem  TreatAsAtomicUnit=on
  Sum : Sum  Inputs=|++
  Sum1 : Sum  Inputs=|-+  SaturateOnIntegerOverflow=on
  Switch : Switch  Criteria=u2 > Threshold
  Switch1 : Switch  Criteria=u2 > Threshold  Threshold=0.5
  Switch2 : Switch  Threshold=0.5
  Switch3 : Switch  Threshold=0.5
  motorC : Subsystem
  P_C : Outport
  wires:
  Switch3/1 -> Outputs to Amplifier/1(Motor current [A])
  Position Measurement/2(Position [m]) -> MATLAB Function1/4(measured_position), Init_motion/1(current_pos), P_C/1, Sum1/1
  Position Measurement/1(init_current) -> Switch3/1
  Switch2/1 -> Sum/1
  CloseLoop_disable/1 -> Switch3/2
  Sum1/1 -> motorC/1(Input)
  Constant/1 -> Switch2/1
  controller_disable/1 -> Switch2/2
  P_C_ref/1 -> Switch/3
  Init/1 -> Position Measurement/1(Init)
  motorC/1(Output) -> Switch2/3
  1_to_enable_id/1 -> Multisine/1(enable)
  "Enable_ID_C "/1 -> Multisine1/1(enable)
  Sum/1 -> Switch3/3
  Multisine1/1(y) -> Sum/2
  Constant4/1 -> Init_motion/2(Init_value)
  1_no_0_init_motion/1 -> Init_motion/3(Switch_to_motion)
  ? -> Init_motion/4(enable_start)
  Switch/1 -> Sum1/2
  enable_refC/1 -> Switch/2
  Constant2/1 -> MATLAB Function1/2(end_time)
  Switch1/1 -> MATLAB Function1/1(reference_end)
  Constant1/1 -> MATLAB Function1/3(Ts)
  MATLAB Function1/1(path) -> Switch/1
  quintic_ref/1 -> Switch1/3
  Constant3/1 -> Switch1/1
  "enable_quintic "/1 -> Switch1/2

== system Ball_and_Plate_MicroLabBox_student/RTI Data/RTI Data Store ==
  RTI Data Store : Subsystem  mask(RTI_DATA_STORE){}
      mask help:
      | RTI Data Store Block. This block is used by RTI to store internal model dependent data. Deleting this block will result in data loss.
      |
      | NEVER DELETE, COPY, OR MODIFY THIS BLOCK!
      mask Help:
      | RTI Data Store Block. This block is used by RTI to store internal model dependent data. Deleting this block will result in data loss.
      | 
      | NEVER DELETE, COPY, OR MODIFY THIS BLOCK!
      mask Display: text(0.5, 0.5, ' ', 'HorizontalAlignment', 'center');

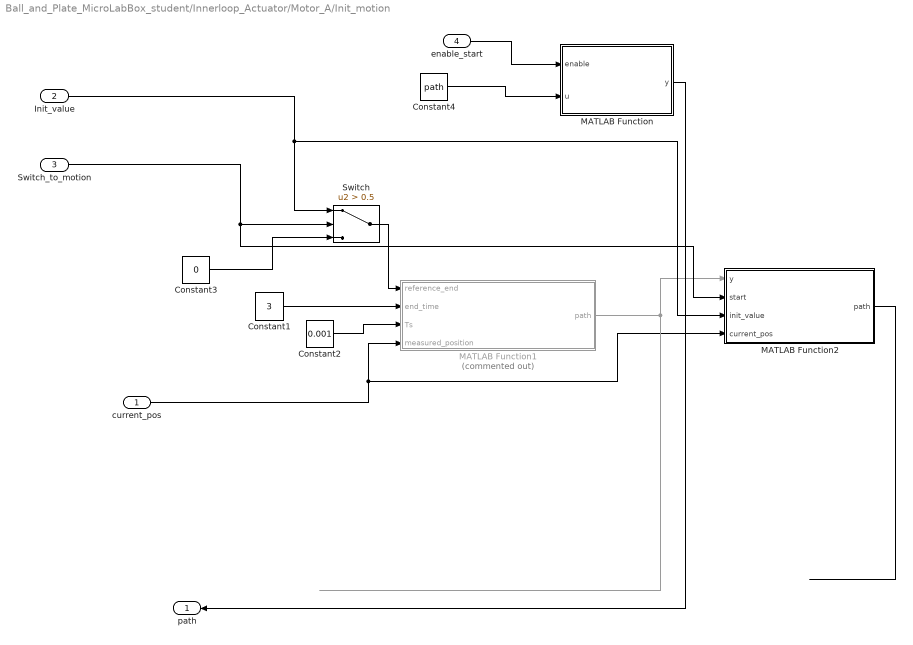
== system Ball_and_Plate_MicroLabBox_student/Innerloop_Actuator/Motor_A/Init_motion ==
  current_pos : Inport
  Init_value : Inport  Port=2
  Switch_to_motion : Inport  Port=3
  "enable_start " : Inport  Port=4
  Constant1 : Constant  Value=3
  Constant2 : Constant  Value=0.001
  Constant3 : Constant  Value=0
  Constant4 : Constant  Value=path
  MATLAB Function : MATLAB Function  TreatAsAtomicUnit=on
  MATLAB Function1 : MATLAB Function  Commented=on  TreatAsAtomicUnit=on
  MATLAB Function2 : MATLAB Function  TreatAsAtomicUnit=on
  Switch : Switch  Criteria=u2 > Threshold  Threshold=0.5
  path : Outport
  wires:
  current_pos/1 -> MATLAB Function2/4(current_pos), MATLAB Function1/4(measured_position)
  MATLAB Function1/1(path) -> MATLAB Function2/1(y)
  Switch_to_motion/1 -> MATLAB Function2/2(start), Switch/2
  Constant3/1 -> Switch/3
  Switch/1 -> MATLAB Function1/1(reference_end)
  Init_value/1 -> Switch/1, MATLAB Function2/3(init_value)
  Constant1/1 -> MATLAB Function1/2(end_time)
  Constant2/1 -> MATLAB Function1/3(Ts)
  MATLAB Function2/1(path) -> ?
  "enable_start "/1 -> MATLAB Function/1(enable)
  Constant4/1 -> MATLAB Function/2(u)
  MATLAB Function/1(y) -> path/1

== system Ball_and_Plate_MicroLabBox_student/Innerloop_Actuator/Motor_A/Multisine ==
  enable : Inport
  Constant : Constant  Value=uA
  MATLAB Function : MATLAB Function  TreatAsAtomicUnit=on
  y : Outport
  wires:
  enable/1 -> MATLAB Function/1(enable)
  MATLAB Function/1(y) -> y/1
  Constant/1 -> MATLAB Function/2(u)

== system Ball_and_Plate_MicroLabBox_student/Innerloop_Actuator/Motor_A/Outputs to Amplifier ==
  Motor current [A] : Inport
  Current2V : Gain  Gain=10/3  SaturateOnIntegerOverflow=on  OutDataTypeStr=Inherit: Same as input  ParamDataTypeStr=Inherit: Same as input
  DAC_CLASS1_BL1 : rti1202lib_dac_class1/DAC_CLASS1_BL1  DSProperties=struct('RTI',struct('Version',uint32(2),'BlockType',struct('isSLSource',uint8(0),'isSLSink',uint8(1),'isHWSource',uint8(0),'isHWSink',uint8(1),'isSetup',uint8(0),'isInline',uint8(1),'isNonInline',uint8(0),'isInterrupt',uint8(0),'isChannelwise',uint8(1)),'IOBoardType',{{'DS120X','STD','DACC1'}},'UnitType','DAC','Identifier','DAC','DialogType','ML','BlockSet','NONE','SlaveProcessor','NONE'))  RTIBlockInterface=struct('InputPortsActive',1,'InputPortsWidth',int32(1),'InputPortsDataType',{{'SS_DOUBLE'}},'InputPortsName',{{['DAC 1']}},'DialogFcn','rti120xstddacc1dacgui','InitLevel',3,'IconTransparency','on','BlockDisplay',{{['DAC CL1\nChannel: 1'],'center'}},'BlockName',struct('Token',{{'DAC_CLASS1_BL1'}}))  RTIBlockParameters=struct('ChannelNo',{{1,'OFF',[]}},'ChannelNumOf',{{1,'OFF',[]}},'InitialValue1',{{'0','OFF',[-10 10]}},'InitialValue2',{{'0','OFF',[-10 10]}},'InitialValue3',{{'0','OFF',[-10 10]}},'InitialValue4',{{'0','OFF',[-10 10]}},'InitialValue5',{{'0','OFF',[-10 10]}},'InitialValue6',{{'0','OFF',[-10 10]}},'InitialValue7',{{'0','OFF',[-10 10]}},'InitialValue8',{{'0','OFF',[-10 10]}},'InitialValue9',{{'0','OFF',[-10 10]}},'InitialValue10',{{'0','OFF',[-10 10]}},'InitialValue11',{{'0','OFF',[-10 10]}},'InitialValue12',{{'0','OFF',[-10 10]}},'InitialValue13',{{'0','OFF',[-10 10]}},'InitialValue14',{{'0','OFF',[-10 10]}},'InitialValue15',{{'0','OFF',[-10 10]}},'InitialValue16',{{'0','OFF',[-10 10]}},'OutputMode',{{ones(1,16),'OFF',[1 2]}},'TermValue1',{{'0','OFF',[-10 10]}},'TermValue2',{{'0','OFF',[-10 10]}},'TermValue3',{{'0','OFF',[-10 10]}},'TermValue4',{{'0','OFF',[-10 10]}},'TermValue5',{{'0','OFF',[-10 10]}},'TermValue6',{{'0','OFF',[-10 10]}},'TermValue7',{{'0','OFF',[-10 10]}},'TermValue8',{{'0','OFF',[-10 10]}},'TermValue9',{{'0','OFF',[-10 10]}},'TermValue10',{{'0','OFF',[-10 10]}},'TermValue11',{{'0','OFF',[-10 10]}},'TermValue12',{{'0','OFF',[-10 10]}},'TermValue13',{{'0','OFF',[-10 10]}},'TermValue14',{{'0','OFF',[-10 10]}},'TermValue15',{{'0','OFF',[-10 10]}},'TermValue16',{{'0','OFF',[-10 10]}},'EnableTermMode',{{0,'OFF',[0 1]}},'TLCFileName',{{'rti120xdac_c1_dac','OFF',[]}},'InitialValueBuildCheck1',{{1,'OFF',[]}},'InitialValueBuildCheck2',{{0,'OFF',[]}},'InitialValueBuildCheck3',{{0,'OFF',[]}},'InitialValueBuildCheck4',{{0,'OFF',[]}},'InitialValueBuildCheck5',{{0,'OFF',[]}},'InitialValueBuildCheck6',{{0,'OFF',[]}},'InitialValueBuildCheck7',{{0,'OFF',[]}},'InitialValueBuildCheck8',{{0,'OFF',[]}},'InitialValueBuildCheck9',{{0,'OFF',[]}},'InitialValueBuildCheck10',{{0,'OFF',[]}},'InitialValueBuildCheck11',{{0,'OFF',[]}},'InitialValueBuildCheck12',{{0,'OFF',[]}},'InitialValueBuildCheck13',{{0,'OFF',[]}},'InitialValueBuildCheck14',{{0,'OFF',[]}},'InitialValueBuildCheck15',{{0,'OFF',[]}},'InitialValueBuildCheck16',{{0,'OFF',[]}},'TermValueBuildCheck1',{{0,'OFF',[]}},'TermValueBuildCheck2',{{0,'OFF',[]}},'TermValueBuildCheck3',{{0,'OFF',[]}},'TermValueBuildCheck4',{{0,'OFF',[]}},'TermValueBuildCheck5',{{0,'OFF',[]}},'TermValueBuildCheck6',{{0,'OFF',[]}},'TermValueBuildCheck7',{{0,'OFF',[]}},'TermValueBuildCheck8',{{0,'OFF',[]}},'TermValueBuildCheck9',{{0,'OFF',[]}},'TermValueBuildCheck10',{{0,'OFF',[]}},'TermValueBuildCheck11',{{0,'OFF',[]}},'TermValueBuildCheck12',{{0,'OFF',[]}},'TermValueBuildCheck13',{{0,'OFF',[]}},'TermValueBuildCheck14',{{0,'OFF',[]}},'TermValueBuildCheck15',{{0,'OFF',[]}},'TermValueBuildCheck16',{{0,'OFF',[]}})  RTISFcnParameters=struct('ChannelNo','int16','ChannelNumOf','int16','InitialValue1','double','InitialValue2','double','InitialValue3','double','InitialValue4','double','InitialValue5','double','InitialValue6','double','InitialValue7','double','InitialValue8','double','InitialValue9','double','InitialValue10','double','InitialValue11','double','InitialValue12','double','InitialValue13','double','InitialValue14','double','InitialValue15','double','InitialValue16','double','OutputMode','int16','TermValue1','double','TermValue2','double','TermValue3','double','TermValue4','double','TermValue5','double','TermValue6','double','TermValue7','double','TermValue8','double','TermValue9','double','TermValue10','double','TermValue11','double','TermValue12','double','TermValue13','double','TermValue14','double','TermValue15','double','TermValue16','double','EnableTermMode','int16','TLCFileName','char')  RTIBlockParaDefault=struct('ChannelNo',1,'ChannelNumOf',1,'InitialValue1',0,'InitialValue2',0,'InitialValue3',0,'InitialValue4',0,'InitialValue5',0,'InitialValue6',0,'InitialValue7',0,'InitialValue8',0,'InitialValue9',0,'InitialValue10',0,'InitialValue11',0,'InitialValue12',0,'InitialValue13',0,'InitialValue14',0,'InitialValue15',0,'InitialValue16',0,'OutputMode',ones(1,16),'TermValue1',0,'TermValue2',0,'TermValue3',0,'TermValue4',0,'TermValue5',0,'TermValue6',0,'TermValue7',0,'TermValue8',0,'TermValue9',0,'TermValue10',0,'TermValue11',0,'TermValue12',0,'TermValue13',0,'TermValue14',0,'TermValue15',0,'TermValue16',0,'EnableTermMode',0,'TLCFileName','rti120xdac_c1_dac','InitialValueBuildCheck1',0,'InitialValueBuildCheck2',0,'InitialValueBuildCheck3',0,'InitialValueBuildCheck4',0,'InitialValueBuildCheck5',0,'InitialValueBuildCheck6',0,'InitialValueBuildCheck7',0,'InitialValueBuildCheck8',0,'InitialValueBuildCheck9',0,'InitialValueBuildCheck10',0,'InitialValueBuildCheck11',0,'InitialValueBuildCheck12',0,'InitialValueBuildCheck13',0,'InitialValueBuildCheck14',0,'InitialValueBuildCheck15',0,'InitialValueBuildCheck16',0,'TermValueBuildCheck1',0,'TermValueBuildCheck2',0,'TermValueBuildCheck3',0,'TermValueBuildCheck4',0,'TermValueBuildCheck5',0,'TermValueBuildCheck6',0,'TermValueBuildCheck7',0,'TermValueBuildCheck8',0,'TermValueBuildCheck9',0,'TermValueBuildCheck10',0,'TermValueBuildCheck11',0,'TermValueBuildCheck12',0,'TermValueBuildCheck13',0,'TermValueBuildCheck14',0,'TermValueBuildCheck15',0,'TermValueBuildCheck16',0)
  DSPscale : Gain  Gain=1/10  SaturateOnIntegerOverflow=on  OutDataTypeStr=Inherit: Same as input  ParamDataTypeStr=Inherit: Same as input
  Saturation : Saturate  UpperLimit=3  LowerLimit=-3
  wires:
  Saturation/1 -> Current2V/1
  Current2V/1 -> DSPscale/1
  Motor current [A]/1 -> Saturation/1
  DSPscale/1 -> DAC_CLASS1_BL1/1

== system Ball_and_Plate_MicroLabBox_student/Innerloop_Actuator/Motor_A/PDcontroller ==
  Input : Inport
  Dct1lowpass3 : S-Function  FunctionName=dlowpass1  Parameters=f_den, 0.001  SFunctionDeploymentMode=off  EnableBusSupport=off  mask(dctools){f_den=300}
      mask prompts: f_den "Pole [Hz]"
      mask help: This block implements a discrete time 1st order lowpass filter.
      mask Display: disp('DCT 1st order lowpass')
  Dctpd2 : S-Function  FunctionName=dpd  Parameters=kp, kv, 0.001  SFunctionDeploymentMode=off  EnableBusSupport=off  mask(dctools){kp=2, kv=3}
      mask help: This block implements a discrete time pd filter.
      mask Display: disp('DCT pd')
  Gain1 : Gain  SaturateOnIntegerOverflow=on  OutDataTypeStr=Inherit: Same as input  ParamDataTypeStr=Inherit: Same as input
  Output : Outport
  wires:
  Input/1 -> Gain1/1
  Gain1/1 -> Dctpd2/1
  Dctpd2/1 -> Dct1lowpass3/1
  Dct1lowpass3/1 -> Output/1
